simulink model "two_phase_PMSM"  (R2017b)
settings: Solver=VariableStepAuto  StartTime=0.0  StopTime=100  RelTol=1e-3
undefined symbols (not defined in the file): J, Lsd, Lsq, M, psi_f, Rs, Z
settings Model: Creator=Алексей  LastModifiedBy=Алексей

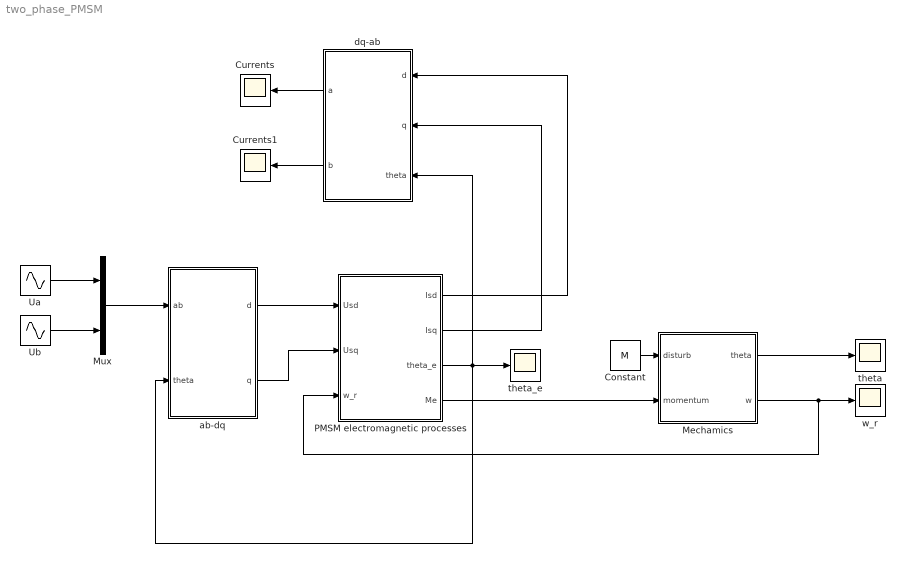
== system two_phase_PMSM ==
  Constant : Constant  Value=M
  Currents : Scope
  Currents1 : Scope
  Mechamics : Subsystem
  Mux : Mux  Inputs=2
  PMSM electromagnetic processes : Subsystem
  Ua : Sin  Amplitude=50  Frequency=50  SampleTime=0
  Ub : Sin  Amplitude=50  Frequency=50  Phase=pi/2  SampleTime=0
  ab-dq : MATLAB Function  TreatAsAtomicUnit=on
  dq-ab : MATLAB Function  TreatAsAtomicUnit=on
  theta : Scope
  theta_e : Scope
  w_r : Scope
  wires:
  Constant/1 -> Mechamics/1(disturb)
  PMSM electromagnetic processes/4(Me) -> Mechamics/2(momentum)
  Mechamics/2(w) -> w_r/1, PMSM electromagnetic processes/3(w_r)
  Mechamics/1(theta) -> theta/1
  PMSM electromagnetic processes/3(theta_e) -> ab-dq/2(theta), dq-ab/3(theta), theta_e/1
  Ua/1 -> Mux/1
  Ub/1 -> Mux/2
  Mux/1 -> ab-dq/1(ab)
  ab-dq/1(d) -> PMSM electromagnetic processes/1(Usd)
  ab-dq/2(q) -> PMSM electromagnetic processes/2(Usq)
  PMSM electromagnetic processes/1(Isd) -> dq-ab/1(d)
  PMSM electromagnetic processes/2(Isq) -> dq-ab/2(q)
  dq-ab/1(a) -> Currents/1
  dq-ab/2(b) -> Currents1/1

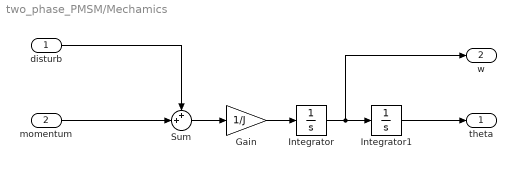
== system two_phase_PMSM/Mechamics ==
  disturb : Inport
  momentum : Inport  Port=2
  Gain : Gain  Gain=1/J
  Integrator : Integrator
  Integrator1 : Integrator
  Sum : Sum  Inputs=++|
  theta : Outport
  w : Outport  Port=2
  wires:
  Integrator/1 -> w/1, Integrator1/1
  disturb/1 -> Sum/1
  momentum/1 -> Sum/2
  Integrator1/1 -> theta/1
  Sum/1 -> Gain/1
  Gain/1 -> Integrator/1

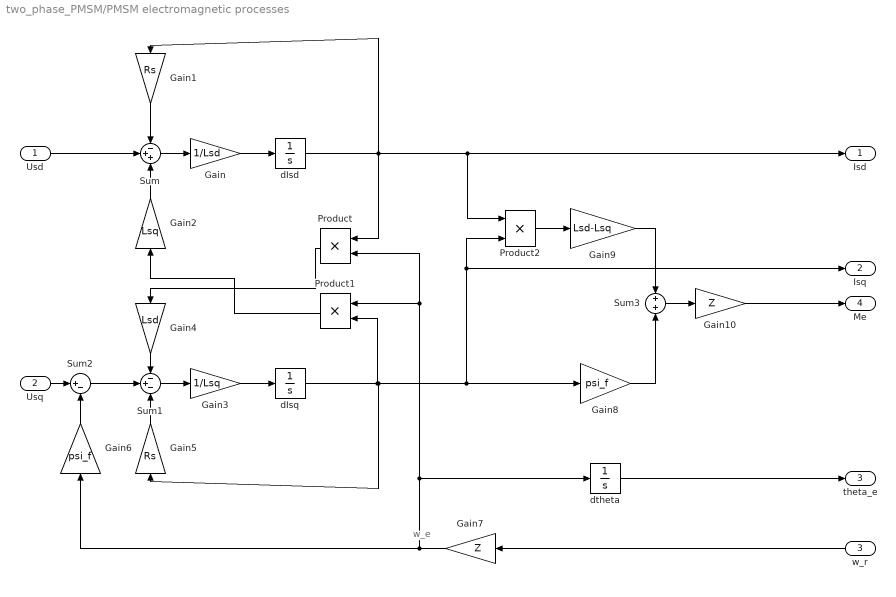
== system two_phase_PMSM/PMSM electromagnetic processes ==
  note: w_e
  Usd : Inport
  Usq : Inport  Port=2
  w_r : Inport  Port=3
  Gain : Gain  Gain=1/Lsd
  Gain1 : Gain  Gain=Rs
  Gain10 : Gain  Gain=Z
  Gain2 : Gain  Gain=Lsq
  Gain3 : Gain  Gain=1/Lsq
  Gain4 : Gain  Gain=Lsd
  Gain5 : Gain  Gain=Rs
  Gain6 : Gain  Gain=psi_f
  Gain7 : Gain  Gain=Z
  Gain8 : Gain  Gain=psi_f
  Gain9 : Gain  Gain=Lsd-Lsq
  Product : Product
  Product1 : Product
  Product2 : Product
  Sum : Sum  Inputs=-++
  Sum1 : Sum  Inputs=-+-
  Sum2 : Sum  Inputs=|+-
  Sum3 : Sum
  dIsd : Integrator
  dIsq : Integrator
  dtheta : Integrator
  Isd : Outport
  Isq : Outport  Port=2
  theta_e : Outport  Port=3
  Me : Outport  Port=4
  wires:
  dtheta/1 -> theta_e/1
  w_r/1 -> Gain7/1
  Usd/1 -> Sum/2
  Usq/1 -> Sum2/1
  Gain10/1 -> Me/1
  Gain8/1 -> Sum3/2
  Gain7/1 -> dtheta/1, Product1/1, Product/2, Gain6/1
  Product2/1 -> Gain9/1
  Product1/1 -> Gain2/1
  dIsd/1 -> Isd/1, Product2/1, Product/1, Gain1/1
  Gain/1 -> dIsd/1
  Gain1/1 -> Sum/1
  Sum3/1 -> Gain10/1
  Gain5/1 -> Sum1/3
  Sum/1 -> Gain/1
  Gain2/1 -> Sum/3
  dIsq/1 -> Product1/2, Gain8/1, Product2/2, Isq/1, Gain5/1
  Gain9/1 -> Sum3/1
  Gain6/1 -> Sum2/2
  Product/1 -> Gain4/1
  Gain3/1 -> dIsq/1
  Sum1/1 -> Gain3/1
  Sum2/1 -> Sum1/2
  Gain4/1 -> Sum1/1

== matlab function two_phase_PMSM/dq-ab ==
  data: d input; q input; a output; theta input; b output
function [a, b] = dq_ab(d, q, theta)
a = d*cos(theta)-q*sin(theta);
b = d*sin(theta)+q*cos(theta);

== matlab function two_phase_PMSM/ab-dq ==
  data: ab input; d output; theta input; q output
function [d, q] = ABC_dq(ab, theta)
a = ab(1);
b = ab(2);

d = b*sin(theta)+a*cos(theta);
q = b*cos(theta)-a*sin(theta);
